simulink model "Template_v4_1_0_2024b_Jetson"  (R2024b)
settings: Solver=ode4  StartTime=0.0  StopTime=tsim  FixedStep=baseRate  RelTol=1e-6  AbsTol=1e-6
undefined symbols (not defined in the file): a1, a2, a3, b0, b1, b2, b3, baseRate, dataRate, DiscIntNeverNeededParam, drop_states_ARM, drop_states_BLACK, drop_states_BLUE, drop_states_RED, F_black_X_nominal, F_black_Y_nominal, F_blue_X_nominal, F_blue_Y_nominal, F_red_X_nominal, F_red_Y_nominal, F_thrusters_BLACK, F_thrusters_BLUE, F_thrusters_RED, Gamma1_el, Gamma1_sh, Gamma1_wr, Gamma2_el, Gamma2_sh, Gamma2_wr, Gamma3_el, Gamma3_sh, Gamma3_wr, Gamma4_el, Gamma4_sh, Gamma4_wr, Gamma5_el, Gamma5_sh, Gamma5_wr, Gamma6_el, Gamma6_sh, Gamma6_wr, home_states_BLACK, home_states_BLUE, home_states_RED, IBLACK, IBLUE, IDIST, IEE, init_states_BLACK, init_states_BLUE, init_states_RED, IPROX, IRED, K_BLACK, K_BLUE, K_RED, Kd_elarm, Kd_sharm, Kd_tb, Kd_tblue ... (+49)
libraries: simulink x30, dspsigops x12, nvidiaSharedBlocks x12, MainLibrary x5, dspinverses x3, nvidiaIMUSensorslib x1
(part 2 of 7)

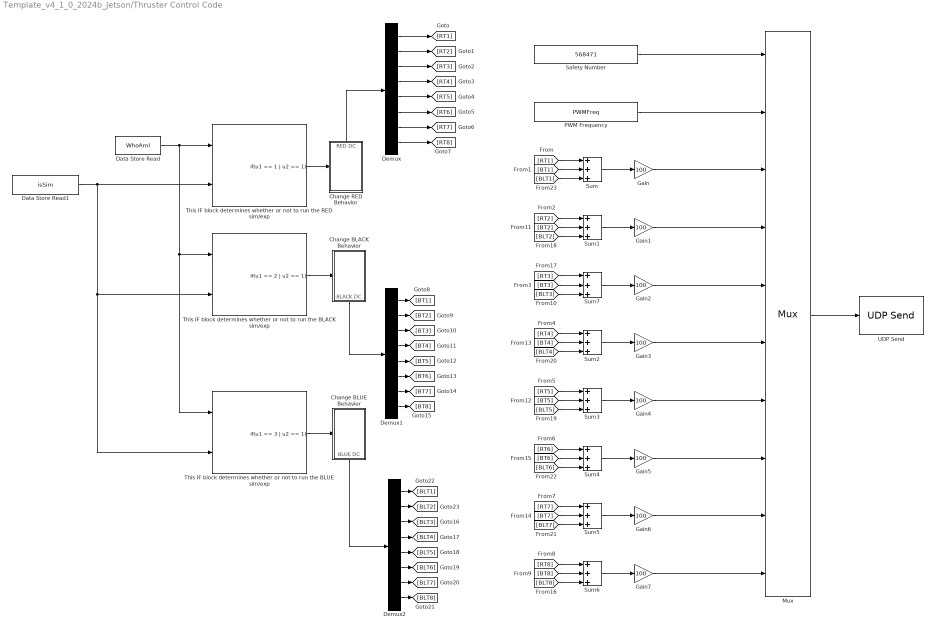
== system Template_v4_1_0_2024b_Jetson/Thruster Control Code ==
  Change BLACK Behavior : Subsystem  TreatAsAtomicUnit=on
  Change BLUE Behavior : Subsystem  TreatAsAtomicUnit=on
  Change RED Behavior : Subsystem  TreatAsAtomicUnit=on
  Data Store Read : DataStoreRead  DataStoreName=WhoAmI  IndexOptions=Index vector (dialog)  Indices=1  OutputSizes=1
  Data Store Read1 : DataStoreRead  DataStoreName=isSim  IndexOptions=Index vector (dialog)  Indices=1  OutputSizes=1
  Demux : Demux  Outputs=8
  Demux1 : Demux  Outputs=8
  Demux2 : Demux  Outputs=8
  Gain{,1..7} (8 alike) : Gain  Gain=100
  Mux : Mux  Inputs=10
  PWM Frequency : Constant  Value=PWMFreq
  Safety Number : Constant  Value=568471
  Sum{,1..7} (8 alike) : Sum  Inputs=+++
  This IF block determines whether or not to run the BLACK sim/exp : If  NumInputs=2  IfExpression=u1 == 2 | u2 == 1  ShowElse=off
  This IF block determines whether or not to run the BLUE sim/exp : If  NumInputs=2  IfExpression=u1 == 3 | u2 == 1  ShowElse=off
  "This IF block determines whether or not to run the RED sim/exp " : If  NumInputs=2  IfExpression=u1 == 1 | u2 == 1  ShowElse=off
  UDP Send : nvidiaSharedBlocks/UDP Send  remoteURL='127.0.0.1'  remotePort=48291  localURL='0.0.0.0'  localPortSource=Automatically determine  localPort=-1  sampletime=-1  blockPlatform=NVIDIA  separateLengthPort=0
      settings: LibrarySourceBlock=nvidiaNetworklib/UDP Send
  wires:
  Data Store Read1/1 -> This IF block determines whether or not to run the BLACK sim/exp/2, This IF block determines whether or not to run the BLUE sim/exp/2, "This IF block determines whether or not to run the RED sim/exp "/2
  "This IF block determines whether or not to run the RED sim/exp "/1 -> Change RED Behavior/Action
  This IF block determines whether or not to run the BLACK sim/exp/1 -> Change BLACK Behavior/Action
  Change RED Behavior/1(RED DC) -> Demux/1
  Demux/1 -> [RT1]
  Demux/2 -> [RT2]
  Demux/3 -> [RT3]
  Demux/4 -> [RT4]
  Demux/5 -> [RT5]
  Demux/6 -> [RT6]
  Demux/7 -> [RT7]
  Demux/8 -> [RT8]
  Demux1/5 -> [BT5]
  Demux1/4 -> [BT4]
  Demux1/1 -> [BT1]
  Demux1/8 -> [BT8]
  Demux1/2 -> [BT2]
  Demux1/7 -> [BT7]
  Demux1/6 -> [BT6]
  Demux1/3 -> [BT3]
  Change BLACK Behavior/1(BLACK DC) -> Demux1/1
  Data Store Read/1 -> This IF block determines whether or not to run the BLUE sim/exp/1, This IF block determines whether or not to run the BLACK sim/exp/1, "This IF block determines whether or not to run the RED sim/exp "/1
  This IF block determines whether or not to run the BLUE sim/exp/1 -> Change BLUE Behavior/Action
  Demux2/5 -> [BLT5]
  Demux2/8 -> [BLT8]
  Demux2/7 -> [BLT7]
  Demux2/2 -> [BLT2]
  Change BLUE Behavior/1(BLUE DC) -> Demux2/1
  Demux2/1 -> [BLT1]
  Demux2/4 -> [BLT4]
  Demux2/3 -> [BLT3]
  Demux2/6 -> [BLT6]
  [BT5] -> Sum3/2
  [RT4] -> Sum2/1
  Sum3/1 -> Gain4/1
  [RT2] -> Sum1/1
  [BLT4] -> Sum2/3
  [BT3] -> Sum7/2
  [RT5] -> Sum3/1
  PWM Frequency/1 -> Mux/2
  Gain3/1 -> Mux/6
  [BT8] -> Sum6/2
  Gain7/1 -> Mux/10
  Sum6/1 -> Gain7/1
  Sum7/1 -> Gain2/1
  [BT4] -> Sum2/2
  [RT7] -> Sum5/1
  [BLT3] -> Sum7/3
  Gain1/1 -> Mux/4
  Gain/1 -> Mux/3
  [BLT5] -> Sum3/3
  Sum1/1 -> Gain1/1
  Sum2/1 -> Gain3/1
  Gain4/1 -> Mux/7
  [BLT6] -> Sum4/3
  [BT6] -> Sum4/2
  [BT2] -> Sum1/2
  [BLT2] -> Sum1/3
  [RT1] -> Sum/1
  Sum/1 -> Gain/1
  [BT7] -> Sum5/2
  Gain6/1 -> Mux/9
  [BLT7] -> Sum5/3
  [RT8] -> Sum6/1
  [RT6] -> Sum4/1
  Mux/1 -> UDP Send/1
  [BLT8] -> Sum6/3
  [BT1] -> Sum/2
  Sum5/1 -> Gain6/1
  Gain5/1 -> Mux/8
  Sum4/1 -> Gain5/1
  [BLT1] -> Sum/3
  Safety Number/1 -> Mux/1
  [RT3] -> Sum7/1
  Gain2/1 -> Mux/5

== system Template_v4_1_0_2024b_Jetson/1 - Experiment Logic/Phase #0: Synchronization ==
  note: Setting the RED thrusters to OFF.
  note: Setting the PUCKS for ALL to OFF.
  note: DISABLE ARM Path Planning.
  note: Setting the BLACK thrusters to OFF.
  note: Setting the BLUE thrusters to OFF.
  note: DISABLE RED Path Planning.
  note: DISABLE BLACK Path Planning.
  note: DISABLE BLUE Path Planning.
  note: DISABLE ARM Control.
  Action Port : ActionPort  ActionPortLabel=if(u1 < u2)
  Constant{1..8} (8 alike) : Constant  Value=0
  Data Store Write : DataStoreWrite  DataStoreName=RED_Control_Law_Enabler  IndexOptions=Index vector (dialog)  Indices=1  OutputSizes=1
  Data Store Write1 : DataStoreWrite  DataStoreName=RED_Logger  IndexOptions=Index vector (dialog)  Indices=1  OutputSizes=1
  Data Store Write2 : DataStoreWrite  DataStoreName=BLACK_Control_Law_Enabler  IndexOptions=Index vector (dialog)  Indices=1  OutputSizes=1
  Data Store Write3 : DataStoreWrite  DataStoreName=BLUE_Control_Law_Enabler  IndexOptions=Index vector (dialog)  Indices=1  OutputSizes=1
  Data Store Write4 : DataStoreWrite  DataStoreName=Float_State  IndexOptions=Index vector (dialog)  Indices=1  OutputSizes=1
  Data Store Write5 : DataStoreWrite  DataStoreName=BLUE_Path_Planner_Selection  IndexOptions=Index vector (dialog)  Indices=1  OutputSizes=1
  Data Store Write6 : DataStoreWrite  DataStoreName=BLACK_Path_Planner_Selection  IndexOptions=Index vector (dialog)  Indices=1  OutputSizes=1
  Data Store Write7 : DataStoreWrite  DataStoreName=RED_Path_Planner_Selection  IndexOptions=Index vector (dialog)  Indices=1  OutputSizes=1
  Data Store Write8 : DataStoreWrite  DataStoreName=ARM_Path_Planner_Selection  IndexOptions=Index vector (dialog)  Indices=1  OutputSizes=1
  Data Store Write9 : DataStoreWrite  DataStoreName=ARM_Control_Law_Enabler  IndexOptions=Index vector (dialog)  Indices=1  OutputSizes=1
  Puck State : Constant  Value=0
  String Constant : StringConstant  String="\"Chaser: Running Phase 0\""
  wires:
  Constant4/1 -> Data Store Write8/1
  Puck State/1 -> Data Store Write4/1
  Constant5/1 -> Data Store Write/1
  Constant1/1 -> Data Store Write2/1
  Constant2/1 -> Data Store Write3/1
  Constant3/1 -> Data Store Write7/1
  Constant6/1 -> Data Store Write6/1
  Constant7/1 -> Data Store Write5/1
  Constant8/1 -> Data Store Write9/1
  String Constant/1 -> Data Store Write1/1

== system Template_v4_1_0_2024b_Jetson/1 - Experiment Logic/Phase #1: Start Floating  ==
  note: DISABLE ARM Control.
  note: Setting the BLACK thrusters to OFF.
  note: Setting the PUCKS for ALL to OFF.
  note: DISABLE RED Path Planning.
  note: Setting the RED thrusters to OFF.
  note: Setting the BLUE thrusters to OFF.
  note: DISABLE ARM Path Planning.
  note: DISABLE BLACK Path Planning.
  note: DISABLE BLUE Path Planning.
  Action Port : ActionPort  ActionPortLabel=elseif((u1 < u3 & u1 >= u2))
  Constant{1..8} (8 alike) : Constant  Value=0
  Data Store Write : DataStoreWrite  DataStoreName=RED_Control_Law_Enabler  IndexOptions=Index vector (dialog)  Indices=1  OutputSizes=1
  Data Store Write1 : DataStoreWrite  DataStoreName=RED_Logger  IndexOptions=Index vector (dialog)  Indices=1  OutputSizes=1
  Data Store Write2 : DataStoreWrite  DataStoreName=BLACK_Control_Law_Enabler  IndexOptions=Index vector (dialog)  Indices=1  OutputSizes=1
  Data Store Write3 : DataStoreWrite  DataStoreName=BLUE_Control_Law_Enabler  IndexOptions=Index vector (dialog)  Indices=1  OutputSizes=1
  Data Store Write4 : DataStoreWrite  DataStoreName=Float_State  IndexOptions=Index vector (dialog)  Indices=1  OutputSizes=1
  Data Store Write5 : DataStoreWrite  DataStoreName=BLUE_Path_Planner_Selection  IndexOptions=Index vector (dialog)  Indices=1  OutputSizes=1
  Data Store Write6 : DataStoreWrite  DataStoreName=BLACK_Path_Planner_Selection  IndexOptions=Index vector (dialog)  Indices=1  OutputSizes=1
  Data Store Write7 : DataStoreWrite  DataStoreName=RED_Path_Planner_Selection  IndexOptions=Index vector (dialog)  Indices=1  OutputSizes=1
  Data Store Write8 : DataStoreWrite  DataStoreName=ARM_Path_Planner_Selection  IndexOptions=Index vector (dialog)  Indices=1  OutputSizes=1
  Data Store Write9 : DataStoreWrite  DataStoreName=ARM_Control_Law_Enabler  IndexOptions=Index vector (dialog)  Indices=1  OutputSizes=1
  Puck State : Constant
  String Constant : StringConstant  String="\"Chaser: Running Phase 1\""
  wires:
  Constant7/1 -> Data Store Write5/1
  Constant2/1 -> Data Store Write3/1
  Constant6/1 -> Data Store Write6/1
  Puck State/1 -> Data Store Write4/1
  Constant1/1 -> Data Store Write2/1
  Constant5/1 -> Data Store Write/1
  Constant3/1 -> Data Store Write7/1
  Constant8/1 -> Data Store Write9/1
  Constant4/1 -> Data Store Write8/1
  String Constant/1 -> Data Store Write1/1

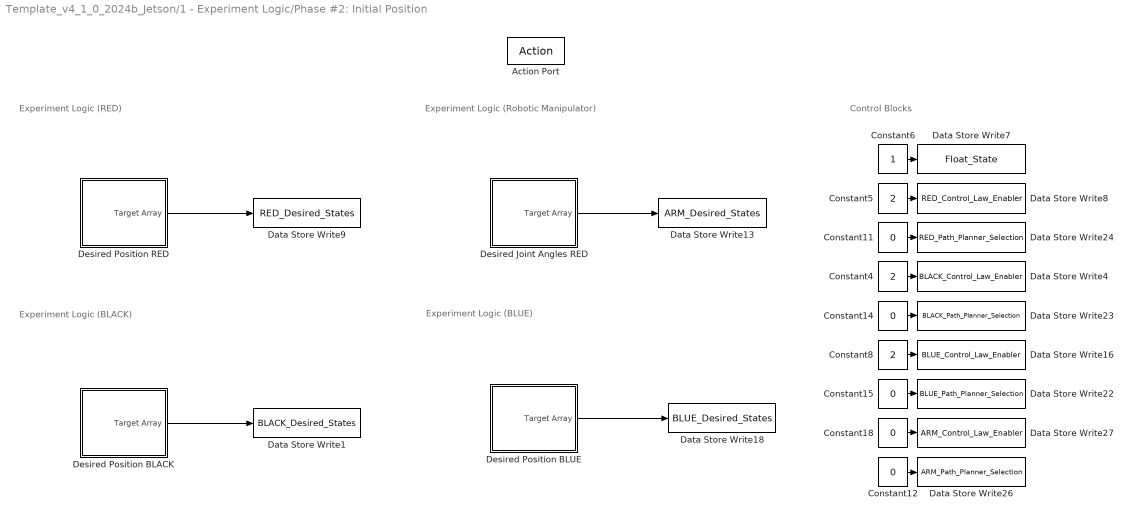
== system Template_v4_1_0_2024b_Jetson/1 - Experiment Logic/Phase #2: Initial Position ==
  note: Experiment Logic (BLACK)
  note: Control Blocks
  note: Experiment Logic (RED)
  note: Experiment Logic (Robotic Manipulator)
  note: Experiment Logic (BLUE)
  Action Port : ActionPort  ActionPortLabel=elseif((u1 < u4 & u1 >= u3))
  Constant{11..12,14..15,18} (5 alike) : Constant  Value=0
  Constant4 : Constant  Value=2
  Constant5 : Constant  Value=2
  Constant6 : Constant
  Constant8 : Constant  Value=2
  Data Store Write1 : DataStoreWrite  DataStoreName=BLACK_Desired_States  IndexOptions=Index vector (dialog)  Indices=1  OutputSizes=1
  Data Store Write13 : DataStoreWrite  DataStoreName=ARM_Desired_States  IndexOptions=Index vector (dialog)  Indices=1  OutputSizes=1
  Data Store Write16 : DataStoreWrite  DataStoreName=BLUE_Control_Law_Enabler  IndexOptions=Index vector (dialog)  Indices=1  OutputSizes=1
  Data Store Write18 : DataStoreWrite  DataStoreName=BLUE_Desired_States  IndexOptions=Index vector (dialog)  Indices=1  OutputSizes=1
  Data Store Write22 : DataStoreWrite  DataStoreName=BLUE_Path_Planner_Selection  IndexOptions=Index vector (dialog)  Indices=1  OutputSizes=1
  Data Store Write23 : DataStoreWrite  DataStoreName=BLACK_Path_Planner_Selection  IndexOptions=Index vector (dialog)  Indices=1  OutputSizes=1
  Data Store Write24 : DataStoreWrite  DataStoreName=RED_Path_Planner_Selection  IndexOptions=Index vector (dialog)  Indices=1  OutputSizes=1
  Data Store Write26 : DataStoreWrite  DataStoreName=ARM_Path_Planner_Selection  IndexOptions=Index vector (dialog)  Indices=1  OutputSizes=1
  Data Store Write27 : DataStoreWrite  DataStoreName=ARM_Control_Law_Enabler  IndexOptions=Index vector (dialog)  Indices=1  OutputSizes=1
  Data Store Write4 : DataStoreWrite  DataStoreName=BLACK_Control_Law_Enabler  IndexOptions=Index vector (dialog)  Indices=1  OutputSizes=1
  Data Store Write7 : DataStoreWrite  DataStoreName=Float_State  IndexOptions=Index vector (dialog)  Indices=1  OutputSizes=1
  Data Store Write8 : DataStoreWrite  DataStoreName=RED_Control_Law_Enabler  IndexOptions=Index vector (dialog)  Indices=1  OutputSizes=1
  Data Store Write9 : DataStoreWrite  DataStoreName=RED_Desired_States  IndexOptions=Index vector (dialog)  Indices=1  OutputSizes=1
  Desired Joint Angles RED : Subsystem
  Desired Position BLACK : Subsystem
  Desired Position BLUE : Subsystem
  Desired Position RED : Subsystem
  wires:
  Constant4/1 -> Data Store Write4/1
  Constant8/1 -> Data Store Write16/1
  Desired Position BLACK/1(Target Array) -> Data Store Write1/1
  Constant5/1 -> Data Store Write8/1
  Desired Position RED/1(Target Array) -> Data Store Write9/1
  Constant6/1 -> Data Store Write7/1
  Desired Position BLUE/1(Target Array) -> Data Store Write18/1
  Constant11/1 -> Data Store Write24/1
  Constant14/1 -> Data Store Write23/1
  Constant15/1 -> Data Store Write22/1
  Desired Joint Angles RED/1(Target Array) -> Data Store Write13/1
  Constant18/1 -> Data Store Write27/1
  Constant12/1 -> Data Store Write26/1

== system Template_v4_1_0_2024b_Jetson/1 - Experiment Logic/Phase #3: Experiment ==
  Action Port : ActionPort  ActionPortLabel=elseif( (u1 < u5 & u1 >= u4))
  Constant1 : Constant  Value=Phase3_SubPhase2_End  SampleTime=-1
  Constant2 : Constant  Value=Phase3_SubPhase3_End  SampleTime=-1
  Constant3 : Constant  Value=Phase3_SubPhase4_End  SampleTime=-1
  Constant4 : Constant  Value=Phase3_SubPhase1_End  SampleTime=-1
  Experiment Sub-Phases : If  NumInputs=5  IfExpression=u1 < u2  ElseIfExpressions=(u1 < u3 & u1 >= u2),(u1 < u4 & u1 >= u3), (u1 < u5 & u1 >= u4)  ShowElse=off
  Sub-Phase #1 : Subsystem  TreatAsAtomicUnit=on
  "Sub-Phase #2 " : Subsystem  TreatAsAtomicUnit=on
  "Sub-Phase #3 " : Subsystem  TreatAsAtomicUnit=on
  Sub-Phase #4 : Subsystem  TreatAsAtomicUnit=on
  Universal_Time : DataStoreRead  DataStoreName=Univ_Time  IndexOptions=Index vector (dialog)  Indices=1  OutputSizes=1
  wires:
  Experiment Sub-Phases/3 -> "Sub-Phase #3 "/Action
  Experiment Sub-Phases/4 -> Sub-Phase #4/Action
  Constant3/1 -> Experiment Sub-Phases/5
  Constant2/1 -> Experiment Sub-Phases/4
  Experiment Sub-Phases/1 -> Sub-Phase #1/Action
  Experiment Sub-Phases/2 -> "Sub-Phase #2 "/Action
  Constant1/1 -> Experiment Sub-Phases/3
  Constant4/1 -> Experiment Sub-Phases/2
  Universal_Time/1 -> Experiment Sub-Phases/1

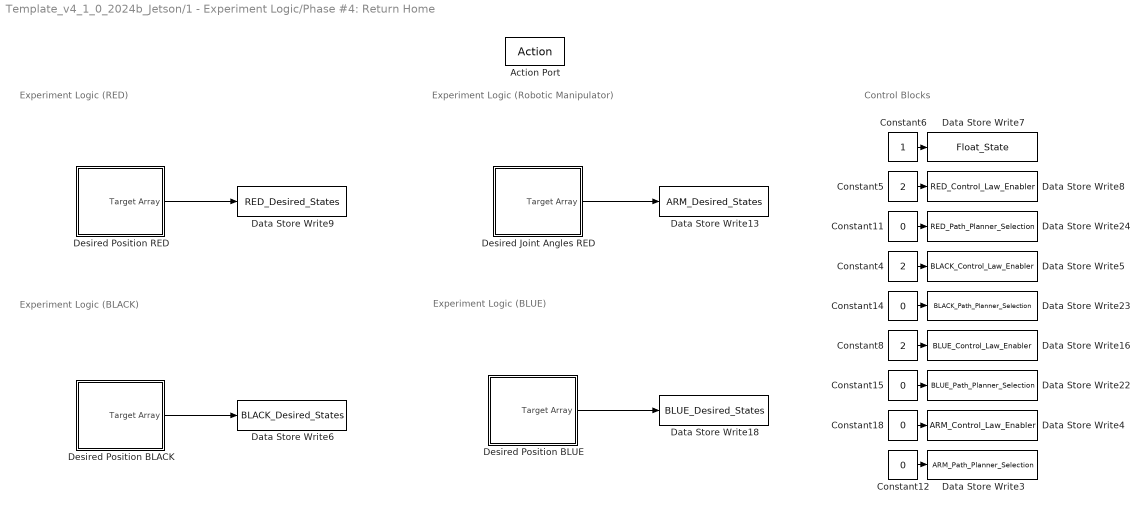
== system Template_v4_1_0_2024b_Jetson/1 - Experiment Logic/Phase #4: Return Home ==
  note: Experiment Logic (BLACK)
  note: Experiment Logic (Robotic Manipulator)
  note: Experiment Logic (BLUE)
  note: Experiment Logic (RED)
  note: Control Blocks
  Action Port : ActionPort  ActionPortLabel=elseif((u1 < u6 & u1 >= u5))
  Constant{11..12,14..15,18} (5 alike) : Constant  Value=0
  Constant4 : Constant  Value=2
  Constant5 : Constant  Value=2
  Constant6 : Constant
  Constant8 : Constant  Value=2
  Data Store Write13 : DataStoreWrite  DataStoreName=ARM_Desired_States  IndexOptions=Index vector (dialog)  Indices=1  OutputSizes=1
  Data Store Write16 : DataStoreWrite  DataStoreName=BLUE_Control_Law_Enabler  IndexOptions=Index vector (dialog)  Indices=1  OutputSizes=1
  Data Store Write18 : DataStoreWrite  DataStoreName=BLUE_Desired_States  IndexOptions=Index vector (dialog)  Indices=1  OutputSizes=1
  Data Store Write22 : DataStoreWrite  DataStoreName=BLUE_Path_Planner_Selection  IndexOptions=Index vector (dialog)  Indices=1  OutputSizes=1
  Data Store Write23 : DataStoreWrite  DataStoreName=BLACK_Path_Planner_Selection  IndexOptions=Index vector (dialog)  Indices=1  OutputSizes=1
  Data Store Write24 : DataStoreWrite  DataStoreName=RED_Path_Planner_Selection  IndexOptions=Index vector (dialog)  Indices=1  OutputSizes=1
  Data Store Write3 : DataStoreWrite  DataStoreName=ARM_Path_Planner_Selection  IndexOptions=Index vector (dialog)  Indices=1  OutputSizes=1
  Data Store Write4 : DataStoreWrite  DataStoreName=ARM_Control_Law_Enabler  IndexOptions=Index vector (dialog)  Indices=1  OutputSizes=1
  Data Store Write5 : DataStoreWrite  DataStoreName=BLACK_Control_Law_Enabler  IndexOptions=Index vector (dialog)  Indices=1  OutputSizes=1
  Data Store Write6 : DataStoreWrite  DataStoreName=BLACK_Desired_States  IndexOptions=Index vector (dialog)  Indices=1  OutputSizes=1
  Data Store Write7 : DataStoreWrite  DataStoreName=Float_State  IndexOptions=Index vector (dialog)  Indices=1  OutputSizes=1
  Data Store Write8 : DataStoreWrite  DataStoreName=RED_Control_Law_Enabler  IndexOptions=Index vector (dialog)  Indices=1  OutputSizes=1
  Data Store Write9 : DataStoreWrite  DataStoreName=RED_Desired_States  IndexOptions=Index vector (dialog)  Indices=1  OutputSizes=1
  Desired Joint Angles RED : Subsystem
  Desired Position BLACK : Subsystem
  Desired Position BLUE : Subsystem
  Desired Position RED : Subsystem
  wires:
  Desired Position RED/1(Target Array) -> Data Store Write9/1
  Desired Position BLACK/1(Target Array) -> Data Store Write6/1
  Desired Position BLUE/1(Target Array) -> Data Store Write18/1
  Constant12/1 -> Data Store Write3/1
  Constant18/1 -> Data Store Write4/1
  Constant6/1 -> Data Store Write7/1
  Constant15/1 -> Data Store Write22/1
  Constant14/1 -> Data Store Write23/1
  Constant5/1 -> Data Store Write8/1
  Constant11/1 -> Data Store Write24/1
  Constant8/1 -> Data Store Write16/1
  Constant4/1 -> Data Store Write5/1
  Desired Joint Angles RED/1(Target Array) -> Data Store Write13/1

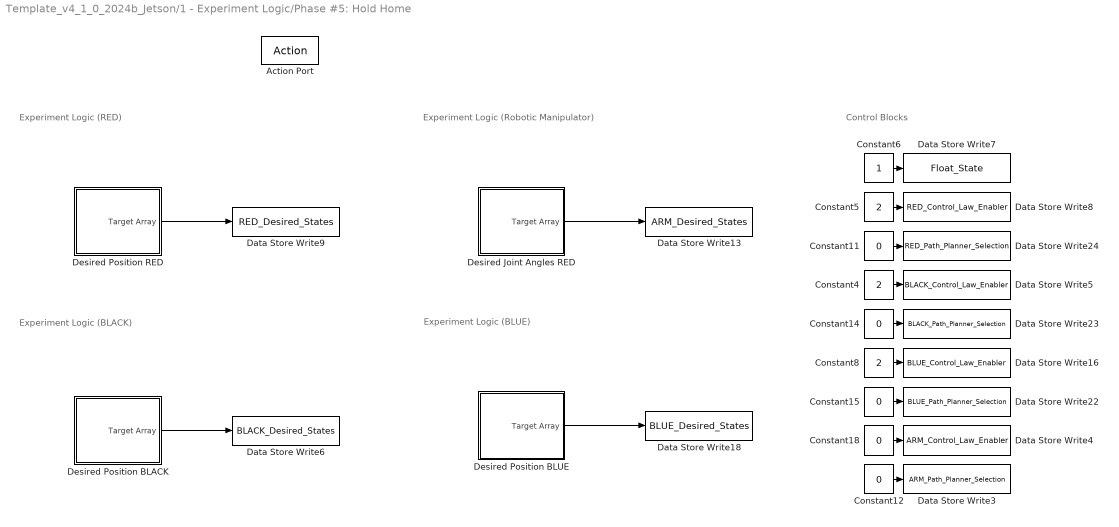
== system Template_v4_1_0_2024b_Jetson/1 - Experiment Logic/Phase #5: Hold Home ==
  note: Experiment Logic (BLUE)
  note: Experiment Logic (BLACK)
  note: Control Blocks
  note: Experiment Logic (RED)
  note: Experiment Logic (Robotic Manipulator)
  Action Port : ActionPort  ActionPortLabel=elseif( (u1 < u7 & u1 >= u6) )
  Constant{11..12,14..15,18} (5 alike) : Constant  Value=0
  Constant4 : Constant  Value=2
  Constant5 : Constant  Value=2
  Constant6 : Constant
  Constant8 : Constant  Value=2
  Data Store Write13 : DataStoreWrite  DataStoreName=ARM_Desired_States  IndexOptions=Index vector (dialog)  Indices=1  OutputSizes=1
  Data Store Write16 : DataStoreWrite  DataStoreName=BLUE_Control_Law_Enabler  IndexOptions=Index vector (dialog)  Indices=1  OutputSizes=1
  Data Store Write18 : DataStoreWrite  DataStoreName=BLUE_Desired_States  IndexOptions=Index vector (dialog)  Indices=1  OutputSizes=1
  Data Store Write22 : DataStoreWrite  DataStoreName=BLUE_Path_Planner_Selection  IndexOptions=Index vector (dialog)  Indices=1  OutputSizes=1
  Data Store Write23 : DataStoreWrite  DataStoreName=BLACK_Path_Planner_Selection  IndexOptions=Index vector (dialog)  Indices=1  OutputSizes=1
  Data Store Write24 : DataStoreWrite  DataStoreName=RED_Path_Planner_Selection  IndexOptions=Index vector (dialog)  Indices=1  OutputSizes=1
  Data Store Write3 : DataStoreWrite  DataStoreName=ARM_Path_Planner_Selection  IndexOptions=Index vector (dialog)  Indices=1  OutputSizes=1
  Data Store Write4 : DataStoreWrite  DataStoreName=ARM_Control_Law_Enabler  IndexOptions=Index vector (dialog)  Indices=1  OutputSizes=1
  Data Store Write5 : DataStoreWrite  DataStoreName=BLACK_Control_Law_Enabler  IndexOptions=Index vector (dialog)  Indices=1  OutputSizes=1
  Data Store Write6 : DataStoreWrite  DataStoreName=BLACK_Desired_States  IndexOptions=Index vector (dialog)  Indices=1  OutputSizes=1
  Data Store Write7 : DataStoreWrite  DataStoreName=Float_State  IndexOptions=Index vector (dialog)  Indices=1  OutputSizes=1
  Data Store Write8 : DataStoreWrite  DataStoreName=RED_Control_Law_Enabler  IndexOptions=Index vector (dialog)  Indices=1  OutputSizes=1
  Data Store Write9 : DataStoreWrite  DataStoreName=RED_Desired_States  IndexOptions=Index vector (dialog)  Indices=1  OutputSizes=1
  Desired Joint Angles RED : Subsystem
  Desired Position BLACK : Subsystem
  Desired Position BLUE : Subsystem
  Desired Position RED : Subsystem
  wires:
  Desired Position RED/1(Target Array) -> Data Store Write9/1
  Desired Position BLACK/1(Target Array) -> Data Store Write6/1
  Desired Position BLUE/1(Target Array) -> Data Store Write18/1
  Constant12/1 -> Data Store Write3/1
  Constant18/1 -> Data Store Write4/1
  Constant6/1 -> Data Store Write7/1
  Constant15/1 -> Data Store Write22/1
  Constant14/1 -> Data Store Write23/1
  Constant5/1 -> Data Store Write8/1
  Constant11/1 -> Data Store Write24/1
  Constant8/1 -> Data Store Write16/1
  Constant4/1 -> Data Store Write5/1
  Desired Joint Angles RED/1(Target Array) -> Data Store Write13/1

== system Template_v4_1_0_2024b_Jetson/1 - Experiment Logic/Phase #6: Clean Shutdown ==
  note: DISABLE ARM Control.
  note: Setting the BLACK thrusters to OFF.
  note: Setting the PUCKS for ALL to OFF.
  note: DISABLE RED Path Planning.
  note: Setting the RED thrusters to OFF.
  note: Setting the BLUE thrusters to OFF.
  note: DISABLE ARM Path Planning.
  note: DISABLE BLACK Path Planning.
  note: DISABLE BLUE Path Planning.
  Action Port : ActionPort  ActionPortLabel=elseif((u1 >= u7))
  Constant{1..8} (8 alike) : Constant  Value=0
  Data Store Write : DataStoreWrite  DataStoreName=RED_Control_Law_Enabler  IndexOptions=Index vector (dialog)  Indices=1  OutputSizes=1
  Data Store Write2 : DataStoreWrite  DataStoreName=BLACK_Control_Law_Enabler  IndexOptions=Index vector (dialog)  Indices=1  OutputSizes=1
  Data Store Write3 : DataStoreWrite  DataStoreName=BLUE_Control_Law_Enabler  IndexOptions=Index vector (dialog)  Indices=1  OutputSizes=1
  Data Store Write4 : DataStoreWrite  DataStoreName=Float_State  IndexOptions=Index vector (dialog)  Indices=1  OutputSizes=1
  Data Store Write5 : DataStoreWrite  DataStoreName=BLUE_Path_Planner_Selection  IndexOptions=Index vector (dialog)  Indices=1  OutputSizes=1
  Data Store Write6 : DataStoreWrite  DataStoreName=BLACK_Path_Planner_Selection  IndexOptions=Index vector (dialog)  Indices=1  OutputSizes=1
  Data Store Write7 : DataStoreWrite  DataStoreName=RED_Path_Planner_Selection  IndexOptions=Index vector (dialog)  Indices=1  OutputSizes=1
  Data Store Write8 : DataStoreWrite  DataStoreName=ARM_Path_Planner_Selection  IndexOptions=Index vector (dialog)  Indices=1  OutputSizes=1
  Data Store Write9 : DataStoreWrite  DataStoreName=ARM_Control_Law_Enabler  IndexOptions=Index vector (dialog)  Indices=1  OutputSizes=1
  Puck State : Constant  Value=0
  wires:
  Constant7/1 -> Data Store Write5/1
  Constant2/1 -> Data Store Write3/1
  Constant6/1 -> Data Store Write6/1
  Puck State/1 -> Data Store Write4/1
  Constant1/1 -> Data Store Write2/1
  Constant5/1 -> Data Store Write/1
  Constant3/1 -> Data Store Write7/1
  Constant8/1 -> Data Store Write9/1
  Constant4/1 -> Data Store Write8/1

== system Template_v4_1_0_2024b_Jetson/2 - Guidance/Custom PPL (ARM) ==
  Action Port : ActionPort  ActionPortLabel=if(u1 == 2)
  Desired Position : Subsystem
  Path : Outport
  wires:
  Desired Position/1(Position Array) -> Path/1

== system Template_v4_1_0_2024b_Jetson/2 - Guidance/Custom PPL (BLACK) ==
  Action Port : ActionPort  ActionPortLabel=elseif(u1 == 2)
  Desired Position : Subsystem
  Path : Outport
  wires:
  Desired Position/1(Position Array) -> Path/1

== system Template_v4_1_0_2024b_Jetson/2 - Guidance/Custom PPL (BLUE) ==
  Action Port : ActionPort  ActionPortLabel=if(u1 == 2)
  Desired Position : Subsystem
  Path : Outport
  wires:
  Desired Position/1(Position Array) -> Path/1

== system Template_v4_1_0_2024b_Jetson/2 - Guidance/Custom PPL (RED) ==
  Action Port : ActionPort  ActionPortLabel=elseif(u1 == 2)
  Desired Position : Subsystem
  Path : Outport
  wires:
  Desired Position/1(Position Array) -> Path/1

== system Template_v4_1_0_2024b_Jetson/2 - Guidance/Default APF PPL (BLACK) ==
  Action Port : ActionPort  ActionPortLabel=if(u1 == 1 )
  Angular Gain : Constant  Value=200
  Attractive Gain : Constant  Value=200
  Current Position RED : Subsystem
  Influence Range : Constant
  MATLAB Function : MATLAB Function  TreatAsAtomicUnit=on
  Obstacles : Subsystem
  RED_Px : DataStoreRead  DataStoreName=BLACK_Desired_States  IndexOptions=Index vector (dialog)  Indices=1  OutputSizes=1
  Repulsive Gain : Constant  Value=5
  Reshape : Reshape  OutputDimensionality=Row vector (2-D)
  Reshape1 : Reshape  OutputDimensionality=Row vector (2-D)
  Path : Outport
  wires:
  Obstacles/1(Obstacle Positions) -> MATLAB Function/3(obstacles)
  MATLAB Function/1(currentPosition) -> Path/1
  Reshape/1 -> MATLAB Function/1(desiredPosition)
  Angular Gain/1 -> MATLAB Function/7(angularGain)
  RED_Px/1 -> Reshape/1
  Attractive Gain/1 -> MATLAB Function/4(attractiveGain)
  Repulsive Gain/1 -> MATLAB Function/5(repulsiveGain)
  Reshape1/1 -> MATLAB Function/2("currentPosition ")
  Influence Range/1 -> MATLAB Function/6(influenceRange)
  Current Position RED/1(Position Array) -> Reshape1/1

== system Template_v4_1_0_2024b_Jetson/2 - Guidance/Default APF PPL (RED) ==
  Action Port : ActionPort  ActionPortLabel=if(u1 == 1 )
  Angular Gain : Constant  Value=200
  Attractive Gain : Constant  Value=200
  Current Position RED : Subsystem
  Influence Range : Constant
  MATLAB Function : MATLAB Function  TreatAsAtomicUnit=on
  Obstacles : Subsystem
  RED_Px : DataStoreRead  DataStoreName=RED_Desired_States  IndexOptions=Index vector (dialog)  Indices=1  OutputSizes=1
  Repulsive Gain : Constant  Value=5
  Reshape : Reshape  OutputDimensionality=Row vector (2-D)
  Reshape1 : Reshape  OutputDimensionality=Row vector (2-D)
  Path : Outport
  wires:
  MATLAB Function/1(currentPosition) -> Path/1
  Reshape/1 -> MATLAB Function/1(desiredPosition)
  Reshape1/1 -> MATLAB Function/2("currentPosition ")
  Current Position RED/1(Position Array) -> Reshape1/1
  Obstacles/1(Obstacle Positions) -> MATLAB Function/3(obstacles)
  RED_Px/1 -> Reshape/1
  Attractive Gain/1 -> MATLAB Function/4(attractiveGain)
  Angular Gain/1 -> MATLAB Function/7(angularGain)
  Influence Range/1 -> MATLAB Function/6(influenceRange)
  Repulsive Gain/1 -> MATLAB Function/5(repulsiveGain)

== system Template_v4_1_0_2024b_Jetson/2 - Guidance/Disable PPL (ARM) ==
  Action Port : ActionPort  ActionPortLabel=else
  Desired Position : Subsystem
  Path : Outport
  wires:
  Desired Position/1(Position Array) -> Path/1

== system Template_v4_1_0_2024b_Jetson/2 - Guidance/Disable PPL (BLACK) ==
  Action Port : ActionPort  ActionPortLabel=else
  Desired Position : Subsystem
  Path : Outport
  wires:
  Desired Position/1(Position Array) -> Path/1

== system Template_v4_1_0_2024b_Jetson/2 - Guidance/Disable PPL (BLUE) ==
  Action Port : ActionPort  ActionPortLabel=else
  Desired Position : Subsystem
  Path : Outport
  wires:
  Desired Position/1(Position Array) -> Path/1

== system Template_v4_1_0_2024b_Jetson/2 - Guidance/Disable PPL (RED) ==
  Action Port : ActionPort  ActionPortLabel=else
  Desired Position : Subsystem
  Path : Outport
  wires:
  Desired Position/1(Position Array) -> Path/1

== system Template_v4_1_0_2024b_Jetson/3 - Control/Custom Control (ARM) ==
  Action Port : ActionPort  ActionPortLabel=elseif(u1 == 2)
  Mux : Mux  Inputs=3
  Zero : Constant  Value=0  OutDataTypeStr=Inherit: Inherit via back propagation
  u : Outport
  wires:
  Mux/1 -> u/1
  Zero/1 -> Mux/3, Mux/1, Mux/2

== system Template_v4_1_0_2024b_Jetson/3 - Control/Custom Control (RED) ==
  Action Port : ActionPort  ActionPortLabel=elseif( u1 == 3)
  Mux : Mux  Inputs=3
  Zero : Constant  Value=0  OutDataTypeStr=Inherit: Inherit via back propagation
  u : Outport
  wires:
  Zero/1 -> Mux/3, Mux/1, Mux/2
  Mux/1 -> u/1

== system Template_v4_1_0_2024b_Jetson/3 - Control/Default LQR Control (BLACK) ==
  Action Port : ActionPort  ActionPortLabel=elseif(u1 == 2)
  Calculate Error : Subsystem
  Constant2 : Constant  Value=-K_BLACK
  Data Store Read1 : DataStoreRead  DataStoreName=BLACK_Path  IndexOptions=Index vector (dialog)  Indices=1  OutputSizes=1
  Data Store Read13 : DataStoreRead  DataStoreName=BLACK_Measured_States  IndexOptions=Index vector (dialog)  Indices=1  OutputSizes=1
  Demux : Demux  Outputs=[1,1,1,1,1,1,3]
  Demux1 : Demux  Outputs=3
  Discrete Derivative : simulink/Discrete/Discrete Derivative  gainval=1.0  ICPrevScaledInput=0.0  OutMin=[]  OutMax=[]  OutDataType=fixdt(1, 16)  OutScaling=2^-10  DoSatur=off
  Discrete Derivative1 : simulink/Discrete/Discrete Derivative  gainval=1.0  ICPrevScaledInput=0.0  OutMin=[]  OutMax=[]  OutDataType=fixdt(1, 16)  OutScaling=2^-10  DoSatur=off
  Discrete Derivative2 : simulink/Discrete/Discrete Derivative  gainval=1.0  ICPrevScaledInput=0.0  OutMin=[]  OutMax=[]  OutDataType=fixdt(1, 16)  OutScaling=2^-10  DoSatur=off
  Matrix Multiply : Product  Multiplication=Matrix(*)
  Mux1 : Mux  Inputs=3
  Mux2 : Mux  Inputs=2
  Mux3 : Mux  Inputs=3
  Reshape1 : Reshape  OutputDimensionality=Column vector (2-D)
  Reshape3 : Reshape  OutputDimensionality=Column vector (2-D)
  Reshape4 : Reshape  OutputDimensionality=Column vector (2-D)
  Subtract{4..8} (5 alike) : Sum  Inputs=-+
  Terminator : Terminator
  u : Outport
  wires:
  Mux2/1 -> Matrix Multiply/2
  Reshape1/1 -> Mux2/1
  Mux1/1 -> Reshape1/1
  Reshape3/1 -> Mux2/2
  Reshape4/1 -> u/1
  Matrix Multiply/1 -> Reshape4/1
  Constant2/1 -> Matrix Multiply/1
  Mux3/1 -> Reshape3/1
  Demux1/2 -> Discrete Derivative1/1, Subtract4/1
  Demux/2 -> Subtract4/2
  Demux1/3 -> Discrete Derivative2/1, Calculate Error/1(Unwrapped Angle)
  Discrete Derivative1/1 -> Subtract6/1
  Demux/4 -> Subtract7/2
  Data Store Read13/1 -> Demux/1
  Demux/1 -> Subtract5/2
  Discrete Derivative/1 -> Subtract7/1
  Data Store Read1/1 -> Demux1/1
  Demux/5 -> Subtract6/2
  Demux/3 -> Calculate Error/2(Unwrapped Angle1)
  Demux/7 -> Terminator/1
  Discrete Derivative2/1 -> Subtract8/1
  Demux1/1 -> Discrete Derivative/1, Subtract5/1
  Demux/6 -> Subtract8/2
  Subtract5/1 -> Mux1/1
  Subtract4/1 -> Mux1/2
  Calculate Error/1(Attitude Error) -> Mux1/3
  Subtract7/1 -> Mux3/1
  Subtract6/1 -> Mux3/2
  Subtract8/1 -> Mux3/3

== system Template_v4_1_0_2024b_Jetson/3 - Control/Default LQR Control (BLUE) ==
  Action Port : ActionPort  ActionPortLabel=elseif(u1 == 2)
  Calculate Error : Subsystem
  Constant2 : Constant  Value=-K_BLUE
  Data Store Read1 : DataStoreRead  DataStoreName=BLUE_Path  IndexOptions=Index vector (dialog)  Indices=1  OutputSizes=1
  Data Store Read2 : DataStoreRead  DataStoreName=BLUE_Measured_States  IndexOptions=Index vector (dialog)  Indices=1  OutputSizes=1
  Demux : Demux  Outputs=[1,1,1,1,1,1,3]
  Demux1 : Demux  Outputs=3
  Discrete Derivative : simulink/Discrete/Discrete Derivative  gainval=1.0  ICPrevScaledInput=0.0  OutMin=[]  OutMax=[]  OutDataType=fixdt(1, 16)  OutScaling=2^-10  DoSatur=off
  Discrete Derivative1 : simulink/Discrete/Discrete Derivative  gainval=1.0  ICPrevScaledInput=0.0  OutMin=[]  OutMax=[]  OutDataType=fixdt(1, 16)  OutScaling=2^-10  DoSatur=off
  Discrete Derivative2 : simulink/Discrete/Discrete Derivative  gainval=1.0  ICPrevScaledInput=0.0  OutMin=[]  OutMax=[]  OutDataType=fixdt(1, 16)  OutScaling=2^-10  DoSatur=off
  Matrix Multiply : Product  Multiplication=Matrix(*)
  Mux : Mux  Inputs=3
  Mux1 : Mux  Inputs=2
  Mux2 : Mux  Inputs=3
  Reshape1 : Reshape  OutputDimensionality=Column vector (2-D)
  Reshape2 : Reshape  OutputDimensionality=Column vector (2-D)
  Reshape4 : Reshape  OutputDimensionality=Column vector (2-D)
  Subtract{4..8} (5 alike) : Sum  Inputs=-+
  Terminator : Terminator
  u : Outport
  wires:
  Calculate Error/1(Attitude Error) -> Mux/3
  Subtract6/1 -> Mux2/2
  Matrix Multiply/1 -> Reshape4/1
  Mux2/1 -> Reshape2/1
  Reshape4/1 -> u/1
  Mux/1 -> Reshape1/1
  Subtract5/1 -> Mux/1
  Reshape2/1 -> Mux1/2
  Mux1/1 -> Matrix Multiply/2
  Subtract7/1 -> Mux2/1
  Constant2/1 -> Matrix Multiply/1
  Subtract4/1 -> Mux/2
  Subtract8/1 -> Mux2/3
  Reshape1/1 -> Mux1/1
  Demux/2 -> Subtract4/2
  Demux/4 -> Subtract7/2
  Demux/7 -> Terminator/1
  Demux/1 -> Subtract5/2
  Data Store Read1/1 -> Demux1/1
  Discrete Derivative2/1 -> Subtract8/1
  Demux1/3 -> Discrete Derivative2/1, Calculate Error/1(Unwrapped Angle)
  Discrete Derivative/1 -> Subtract7/1
  Demux/3 -> Calculate Error/2(Unwrapped Angle1)
  Demux1/2 -> Discrete Derivative1/1, Subtract4/1
  Demux/6 -> Subtract8/2
  Demux/5 -> Subtract6/2
  Data Store Read2/1 -> Demux/1
  Demux1/1 -> Discrete Derivative/1, Subtract5/1
  Discrete Derivative1/1 -> Subtract6/1

== system Template_v4_1_0_2024b_Jetson/3 - Control/Default LQR Control (RED) ==
  Action Port : ActionPort  ActionPortLabel=elseif(u1 == 2)
  Calculate Error : Subsystem
  Constant2 : Constant  Value=-K_RED
  Data Store Read1 : DataStoreRead  DataStoreName=RED_Path  IndexOptions=Index vector (dialog)  Indices=1  OutputSizes=1
  Data Store Read13 : DataStoreRead  DataStoreName=RED_Measured_States  IndexOptions=Index vector (dialog)  Indices=1  OutputSizes=1
  Demux : Demux  Outputs=[1,1,1,1,1,1,3]
  Demux1 : Demux  Outputs=3
  Discrete Derivative : simulink/Discrete/Discrete Derivative  gainval=1.0  ICPrevScaledInput=0.0  OutMin=[]  OutMax=[]  OutDataType=fixdt(1, 16)  OutScaling=2^-10  DoSatur=off
  Discrete Derivative1 : simulink/Discrete/Discrete Derivative  gainval=1.0  ICPrevScaledInput=0.0  OutMin=[]  OutMax=[]  OutDataType=fixdt(1, 16)  OutScaling=2^-10  DoSatur=off
  Discrete Derivative2 : simulink/Discrete/Discrete Derivative  gainval=1.0  ICPrevScaledInput=0.0  OutMin=[]  OutMax=[]  OutDataType=fixdt(1, 16)  OutScaling=2^-10  DoSatur=off
  Display : Display
  Matrix Multiply : Product  Multiplication=Matrix(*)
  Mux1 : Mux  Inputs=3
  Mux2 : Mux  Inputs=2
  Mux3 : Mux  Inputs=3
  Reshape2 : Reshape  OutputDimensionality=Column vector (2-D)
  Reshape3 : Reshape  OutputDimensionality=Column vector (2-D)
  Reshape4 : Reshape  OutputDimensionality=Column vector (2-D)
  Subtract{4..8} (5 alike) : Sum  Inputs=-+
  Terminator : Terminator
  u : Outport
  wires:
  Subtract5/1 -> Mux1/1
  Mux2/1 -> Matrix Multiply/2
  Reshape3/1 -> Mux2/2
  Mux1/1 -> Reshape2/1
  Matrix Multiply/1 -> Reshape4/1
  Reshape4/1 -> u/1
  Subtract7/1 -> Mux3/1
  Reshape2/1 -> Mux2/1
  Mux3/1 -> Reshape3/1
  Constant2/1 -> Matrix Multiply/1
  Subtract4/1 -> Mux1/2
  Subtract8/1 -> Mux3/3
  Calculate Error/1(Attitude Error) -> Mux1/3
  Subtract6/1 -> Mux3/2
  Demux1/1 -> Discrete Derivative/1, Subtract5/1
  Discrete Derivative/1 -> Subtract7/1
  Demux1/3 -> Discrete Derivative2/1, Calculate Error/1(Unwrapped Angle)
  Discrete Derivative1/1 -> Subtract6/1
  Demux/5 -> Subtract6/2
  Demux/3 -> Calculate Error/2(Unwrapped Angle1)
  Demux/7 -> Terminator/1
  Data Store Read1/1 -> Demux1/1
  Demux/2 -> Subtract4/2
  Demux/1 -> Subtract5/2
  Demux/4 -> Subtract7/2
  Demux1/2 -> Discrete Derivative1/1, Subtract4/1
  Discrete Derivative2/1 -> Subtract8/1
  Data Store Read13/1 -> Display/1, Demux/1
  Demux/6 -> Subtract8/2

== system Template_v4_1_0_2024b_Jetson/3 - Control/Default PD (ARM) ==
  Action Port : ActionPort  ActionPortLabel=if(u1 == 1 )
  Constant7 : Constant
  Data Store Read2 : DataStoreRead  DataStoreName=ARM_Path  IndexOptions=Index vector (dialog)  Indices=1  OutputSizes=1
  Data Store Read4 : DataStoreRead  DataStoreName=isSim  IndexOptions=Index vector (dialog)  Indices=1  OutputSizes=1
  Data Store Write12 : DataStoreWrite  DataStoreName=ARM_Control_Mode  IndexOptions=Index vector (dialog)  Indices=1  OutputSizes=1
  Demux : Demux  Outputs=3
  "If 'simMode' set to '1', then this is a simulation and the dynamics will be simulated. Otherwise, this is an experiment, and the simulation will not be run." : If  IfExpression=u1 == 1
  Merge3 : Merge
  Merge4 : Merge
  Merge5 : Merge
  Mux : Mux  Inputs=3
  Passthrough for Experiment : Subsystem  TreatAsAtomicUnit=on
  Scope : Scope
  Simulated Position Controller : Subsystem  TreatAsAtomicUnit=on
  u : Outport
  wires:
  Passthrough for Experiment/3(q3_command) -> Merge5/2
  Data Store Read4/1 -> "If 'simMode' set to '1', then this is a simulation and the dynamics will be simulated. Otherwise, this is an experiment, and the simulation will not be run."/1
  Demux/3 -> Passthrough for Experiment/3(q3_desired), Simulated Position Controller/3(q3_desired)
  Simulated Position Controller/1(q1_command) -> Merge3/1
  Simulated Position Controller/3(q3_command) -> Merge5/1
  "If 'simMode' set to '1', then this is a simulation and the dynamics will be simulated. Otherwise, this is an experiment, and the simulation will not be run."/1 -> Simulated Position Controller/Action
  Demux/2 -> Passthrough for Experiment/2(q2_desired), Simulated Position Controller/2(q2_desired)
  Passthrough for Experiment/2(q2_command) -> Merge4/2
  Simulated Position Controller/2(q2_command) -> Merge4/1
  Constant7/1 -> Data Store Write12/1
  Passthrough for Experiment/1(q1_command) -> Merge3/2
  Demux/1 -> Passthrough for Experiment/1(q1_desired), Simulated Position Controller/1(q1_desired)
  "If 'simMode' set to '1', then this is a simulation and the dynamics will be simulated. Otherwise, this is an experiment, and the simulation will not be run."/2 -> Passthrough for Experiment/Action
  Merge3/1 -> Mux/1
  Merge4/1 -> Mux/2
  Merge5/1 -> Mux/3
  Mux/1 -> Scope/1, u/1
  Data Store Read2/1 -> Demux/1

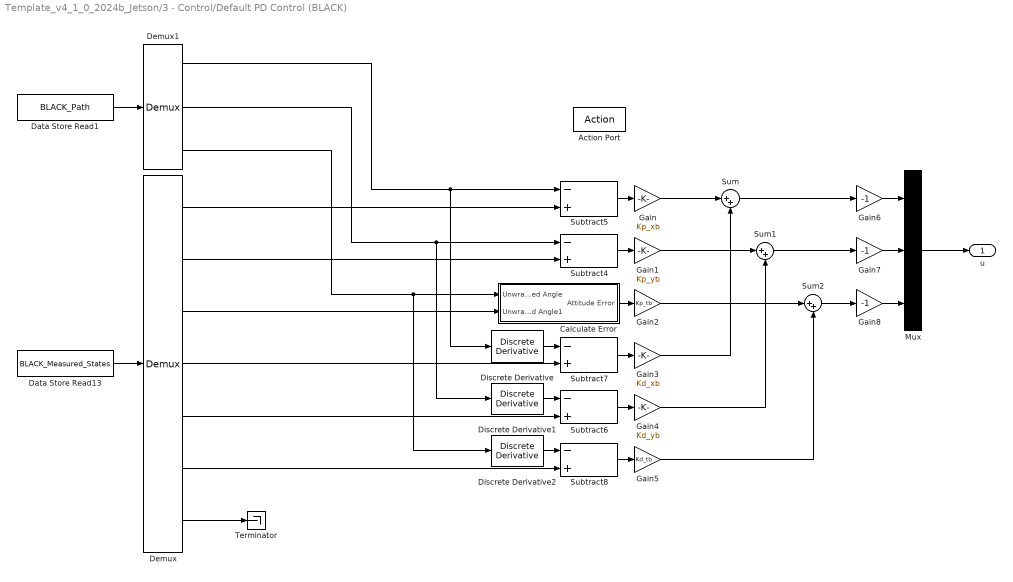
== system Template_v4_1_0_2024b_Jetson/3 - Control/Default PD Control (BLACK) ==
  Action Port : ActionPort  ActionPortLabel=if(u1 == 1 )
  Calculate Error : Subsystem
  Data Store Read1 : DataStoreRead  DataStoreName=BLACK_Path  IndexOptions=Index vector (dialog)  Indices=1  OutputSizes=1
  Data Store Read13 : DataStoreRead  DataStoreName=BLACK_Measured_States  IndexOptions=Index vector (dialog)  Indices=1  OutputSizes=1
  Demux : Demux  Outputs=[1,1,1,1,1,1,3]
  Demux1 : Demux  Outputs=3
  Discrete Derivative : simulink/Discrete/Discrete Derivative  gainval=1.0  ICPrevScaledInput=0.0  OutMin=[]  OutMax=[]  OutDataType=fixdt(1, 16)  OutScaling=2^-10  DoSatur=off
  Discrete Derivative1 : simulink/Discrete/Discrete Derivative  gainval=1.0  ICPrevScaledInput=0.0  OutMin=[]  OutMax=[]  OutDataType=fixdt(1, 16)  OutScaling=2^-10  DoSatur=off
  Discrete Derivative2 : simulink/Discrete/Discrete Derivative  gainval=1.0  ICPrevScaledInput=0.0  OutMin=[]  OutMax=[]  OutDataType=fixdt(1, 16)  OutScaling=2^-10  DoSatur=off
  Gain : Gain  Gain=Kp_xb
  Gain1 : Gain  Gain=Kp_yb
  Gain2 : Gain  Gain=Kp_tb
  Gain3 : Gain  Gain=Kd_xb
  Gain4 : Gain  Gain=Kd_yb
  Gain5 : Gain  Gain=Kd_tb
  Gain6 : Gain  Gain=-1
  Gain7 : Gain  Gain=-1
  Gain8 : Gain  Gain=-1
  Mux : Mux  Inputs=3
  Subtract{4..8} (5 alike) : Sum  Inputs=-+
  Sum : Sum  Inputs=|++
  Sum1 : Sum  Inputs=|++
  Sum2 : Sum  Inputs=|++
  Terminator : Terminator
  u : Outport
  wires:
  Demux/6 -> Subtract8/2
  Subtract8/1 -> Gain5/1
  Gain8/1 -> Mux/3
  Discrete Derivative2/1 -> Subtract8/1
  Gain1/1 -> Sum1/1
  Subtract5/1 -> Gain/1
  Discrete Derivative1/1 -> Subtract6/1
  Subtract6/1 -> Gain4/1
  Demux/2 -> Subtract4/2
  Demux/1 -> Subtract5/2
  Sum1/1 -> Gain7/1
  Demux/4 -> Subtract7/2
  Demux1/3 -> Discrete Derivative2/1, Calculate Error/1(Unwrapped Angle)
  Sum/1 -> Gain6/1
  Subtract4/1 -> Gain1/1
  Demux/3 -> Calculate Error/2(Unwrapped Angle1)
  Subtract7/1 -> Gain3/1
  Gain3/1 -> Sum/2
  Mux/1 -> u/1
  Gain4/1 -> Sum1/2
  Demux1/2 -> Discrete Derivative1/1, Subtract4/1
  Gain/1 -> Sum/1
  Demux/5 -> Subtract6/2
  Gain5/1 -> Sum2/2
  Discrete Derivative/1 -> Subtract7/1
  Demux1/1 -> Discrete Derivative/1, Subtract5/1
  Sum2/1 -> Gain8/1
  Calculate Error/1(Attitude Error) -> Gain2/1
  Gain7/1 -> Mux/2
  Gain6/1 -> Mux/1
  Gain2/1 -> Sum2/1
  Data Store Read13/1 -> Demux/1
  Demux/7 -> Terminator/1
  Data Store Read1/1 -> Demux1/1

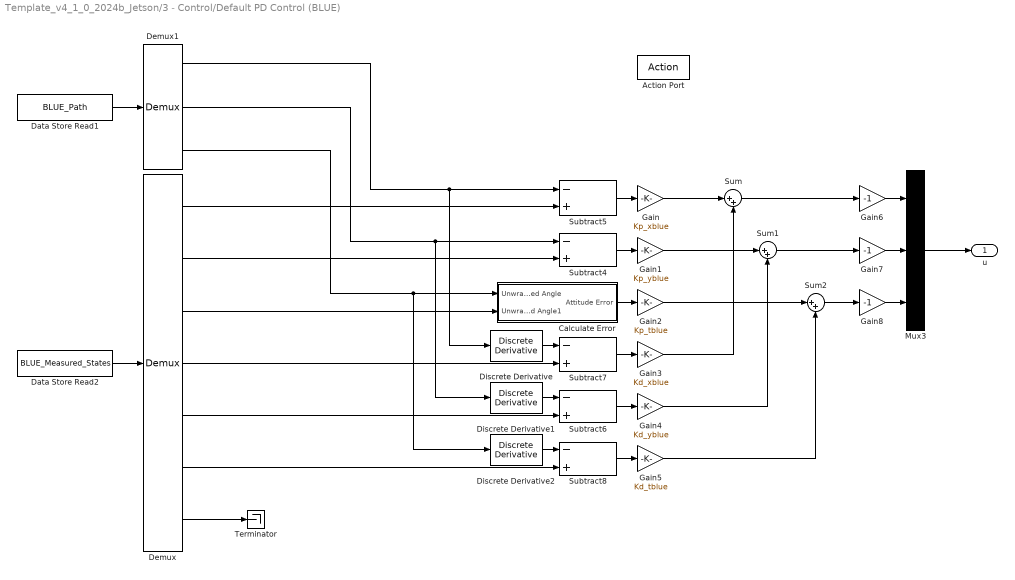
== system Template_v4_1_0_2024b_Jetson/3 - Control/Default PD Control (BLUE) ==
  Action Port : ActionPort  ActionPortLabel=if(u1 == 1 )
  Calculate Error : Subsystem
  Data Store Read1 : DataStoreRead  DataStoreName=BLUE_Path  IndexOptions=Index vector (dialog)  Indices=1  OutputSizes=1
  Data Store Read2 : DataStoreRead  DataStoreName=BLUE_Measured_States  IndexOptions=Index vector (dialog)  Indices=1  OutputSizes=1
  Demux : Demux  Outputs=[1,1,1,1,1,1,3]
  Demux1 : Demux  Outputs=3
  Discrete Derivative : simulink/Discrete/Discrete Derivative  gainval=1.0  ICPrevScaledInput=0.0  OutMin=[]  OutMax=[]  OutDataType=fixdt(1, 16)  OutScaling=2^-10  DoSatur=off
  Discrete Derivative1 : simulink/Discrete/Discrete Derivative  gainval=1.0  ICPrevScaledInput=0.0  OutMin=[]  OutMax=[]  OutDataType=fixdt(1, 16)  OutScaling=2^-10  DoSatur=off
  Discrete Derivative2 : simulink/Discrete/Discrete Derivative  gainval=1.0  ICPrevScaledInput=0.0  OutMin=[]  OutMax=[]  OutDataType=fixdt(1, 16)  OutScaling=2^-10  DoSatur=off
  Gain : Gain  Gain=Kp_xblue
  Gain1 : Gain  Gain=Kp_yblue
  Gain2 : Gain  Gain=Kp_tblue
  Gain3 : Gain  Gain=Kd_xblue
  Gain4 : Gain  Gain=Kd_yblue
  Gain5 : Gain  Gain=Kd_tblue
  Gain6 : Gain  Gain=-1
  Gain7 : Gain  Gain=-1
  Gain8 : Gain  Gain=-1
  Mux3 : Mux  Inputs=3
  Subtract{4..8} (5 alike) : Sum  Inputs=-+
  Sum : Sum  Inputs=|++
  Sum1 : Sum  Inputs=|++
  Sum2 : Sum  Inputs=|++
  Terminator : Terminator
  u : Outport
  wires:
  Sum/1 -> Gain6/1
  Mux3/1 -> u/1
  Gain3/1 -> Sum/2
  Sum2/1 -> Gain8/1
  Gain5/1 -> Sum2/2
  Sum1/1 -> Gain7/1
  Gain6/1 -> Mux3/1
  Gain4/1 -> Sum1/2
  Gain1/1 -> Sum1/1
  Gain2/1 -> Sum2/1
  Gain8/1 -> Mux3/3
  Gain7/1 -> Mux3/2
  Gain/1 -> Sum/1
  Demux1/1 -> Discrete Derivative/1, Subtract5/1
  Discrete Derivative/1 -> Subtract7/1
  Demux1/3 -> Discrete Derivative2/1, Calculate Error/1(Unwrapped Angle)
  Discrete Derivative1/1 -> Subtract6/1
  Demux/5 -> Subtract6/2
  Demux/3 -> Calculate Error/2(Unwrapped Angle1)
  Demux/7 -> Terminator/1
  Data Store Read1/1 -> Demux1/1
  Demux/2 -> Subtract4/2
  Demux/1 -> Subtract5/2
  Demux/4 -> Subtract7/2
  Demux1/2 -> Discrete Derivative1/1, Subtract4/1
  Discrete Derivative2/1 -> Subtract8/1
  Data Store Read2/1 -> Demux/1
  Demux/6 -> Subtract8/2
  Subtract5/1 -> Gain/1
  Subtract4/1 -> Gain1/1
  Calculate Error/1(Attitude Error) -> Gain2/1
  Subtract7/1 -> Gain3/1
  Subtract6/1 -> Gain4/1
  Subtract8/1 -> Gain5/1

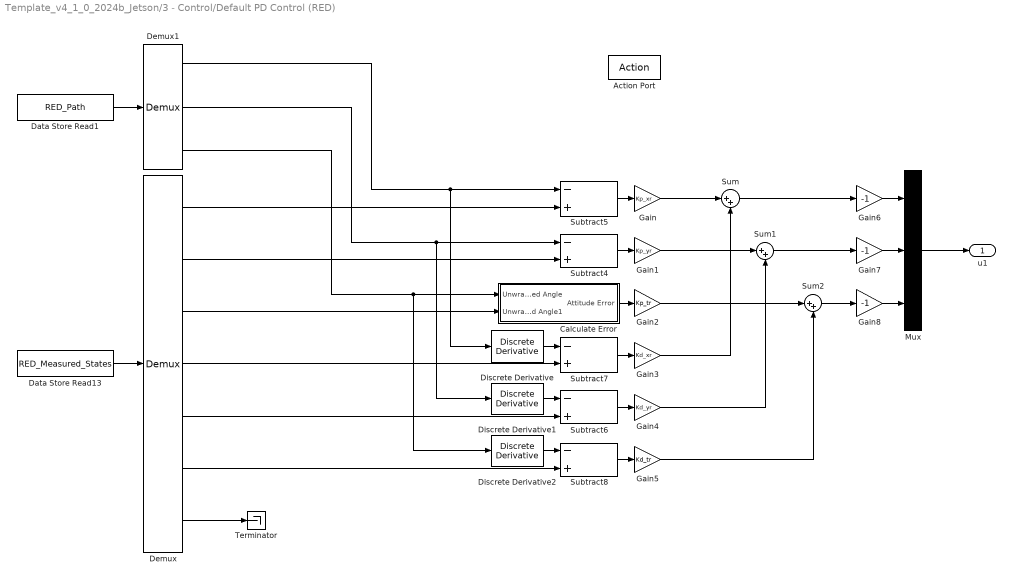
== system Template_v4_1_0_2024b_Jetson/3 - Control/Default PD Control (RED) ==
  Action Port : ActionPort  ActionPortLabel=if(u1 == 1 )
  Calculate Error : Subsystem
  Data Store Read1 : DataStoreRead  DataStoreName=RED_Path  IndexOptions=Index vector (dialog)  Indices=1  OutputSizes=1
  Data Store Read13 : DataStoreRead  DataStoreName=RED_Measured_States  IndexOptions=Index vector (dialog)  Indices=1  OutputSizes=1
  Demux : Demux  Outputs=[1,1,1,1,1,1,3]
  Demux1 : Demux  Outputs=3
  Discrete Derivative : simulink/Discrete/Discrete Derivative  gainval=1.0  ICPrevScaledInput=0.0  OutMin=[]  OutMax=[]  OutDataType=fixdt(1, 16)  OutScaling=2^-10  DoSatur=off
  Discrete Derivative1 : simulink/Discrete/Discrete Derivative  gainval=1.0  ICPrevScaledInput=0.0  OutMin=[]  OutMax=[]  OutDataType=fixdt(1, 16)  OutScaling=2^-10  DoSatur=off
  Discrete Derivative2 : simulink/Discrete/Discrete Derivative  gainval=1.0  ICPrevScaledInput=0.0  OutMin=[]  OutMax=[]  OutDataType=fixdt(1, 16)  OutScaling=2^-10  DoSatur=off
  Gain : Gain  Gain=Kp_xr
  Gain1 : Gain  Gain=Kp_yr
  Gain2 : Gain  Gain=Kp_tr
  Gain3 : Gain  Gain=Kd_xr
  Gain4 : Gain  Gain=Kd_yr
  Gain5 : Gain  Gain=Kd_tr
  Gain6 : Gain  Gain=-1
  Gain7 : Gain  Gain=-1
  Gain8 : Gain  Gain=-1
  Mux : Mux  Inputs=3
  Subtract{4..8} (5 alike) : Sum  Inputs=-+
  Sum : Sum  Inputs=|++
  Sum1 : Sum  Inputs=|++
  Sum2 : Sum  Inputs=|++
  Terminator : Terminator
  u1 : Outport
  wires:
  Gain6/1 -> Mux/1
  Gain8/1 -> Mux/3
  Gain1/1 -> Sum1/1
  Sum/1 -> Gain6/1
  Gain5/1 -> Sum2/2
  Gain3/1 -> Sum/2
  Sum1/1 -> Gain7/1
  Mux/1 -> u1/1
  Gain4/1 -> Sum1/2
  Sum2/1 -> Gain8/1
  Gain/1 -> Sum/1
  Gain7/1 -> Mux/2
  Gain2/1 -> Sum2/1
  Demux1/2 -> Discrete Derivative1/1, Subtract4/1
  Demux/2 -> Subtract4/2
  Demux1/3 -> Discrete Derivative2/1, Calculate Error/1(Unwrapped Angle)
  Discrete Derivative1/1 -> Subtract6/1
  Demux/4 -> Subtract7/2
  Data Store Read13/1 -> Demux/1
  Demux/1 -> Subtract5/2
  Discrete Derivative/1 -> Subtract7/1
  Data Store Read1/1 -> Demux1/1
  Demux/5 -> Subtract6/2
  Demux/3 -> Calculate Error/2(Unwrapped Angle1)
  Demux/7 -> Terminator/1
  Discrete Derivative2/1 -> Subtract8/1
  Demux1/1 -> Discrete Derivative/1, Subtract5/1
  Demux/6 -> Subtract8/2
  Subtract5/1 -> Gain/1
  Subtract4/1 -> Gain1/1
  Calculate Error/1(Attitude Error) -> Gain2/1
  Subtract7/1 -> Gain3/1
  Subtract6/1 -> Gain4/1
  Subtract8/1 -> Gain5/1

== system Template_v4_1_0_2024b_Jetson/3 - Control/Disable Control (ARM) ==
  Action Port : ActionPort  ActionPortLabel=else
  Constant7 : Constant  Value=0
  Data Store Write12 : DataStoreWrite  DataStoreName=ARM_Control_Mode  IndexOptions=Index vector (dialog)  Indices=1  OutputSizes=1
  Mux : Mux  Inputs=3
  Zero : Constant  Value=0  OutDataTypeStr=Inherit: Inherit via back propagation
  Out1 : Outport
  wires:
  Mux/1 -> Out1/1
  Zero/1 -> Mux/3, Mux/1, Mux/2
  Constant7/1 -> Data Store Write12/1

== system Template_v4_1_0_2024b_Jetson/3 - Control/Disable Thrusters (BLACK) ==
  Action Port : ActionPort  ActionPortLabel=else
  Mux : Mux  Inputs=3
  Zero : Constant  Value=0  OutDataTypeStr=Inherit: Inherit via back propagation
  Out1 : Outport
  wires:
  Zero/1 -> Mux/3, Mux/1, Mux/2
  Mux/1 -> Out1/1

== system Template_v4_1_0_2024b_Jetson/3 - Control/Disable Thrusters (BLUE) ==
  Action Port : ActionPort  ActionPortLabel=else
  Mux : Mux  Inputs=3
  Zero : Constant  Value=0  OutDataTypeStr=Inherit: Inherit via back propagation
  Out1 : Outport
  wires:
  Zero/1 -> Mux/3, Mux/1, Mux/2
  Mux/1 -> Out1/1

== system Template_v4_1_0_2024b_Jetson/3 - Control/Disable Thrusters (RED) ==
  Action Port : ActionPort  ActionPortLabel=else
  Mux : Mux  Inputs=3
  Zero : Constant  Value=0  OutDataTypeStr=Inherit: Inherit via back propagation
  u : Outport
  wires:
  Zero/1 -> Mux/3, Mux/1, Mux/2
  Mux/1 -> u/1

== system Template_v4_1_0_2024b_Jetson/Check Connection/Change BLACK Behavior ==
  Action Port : ActionPort  ActionPortLabel=if(u1 == 2 & u2 == 0)
  Constant1 : Constant  OutDataTypeStr=int32
  UDP Send : nvidiaSharedBlocks/UDP Send  remoteURL='255.255.255.255'  remotePort=33002  localURL='0.0.0.0'  localPortSource=Automatically determine  localPort=-1  sampletime=-1  blockPlatform=NVIDIA  separateLengthPort=0
      settings: LibrarySourceBlock=nvidiaNetworklib/UDP Send
  wires:
  Constant1/1 -> UDP Send/1

== system Template_v4_1_0_2024b_Jetson/Check Connection/Change BLUE Behavior ==
  Action Port : ActionPort  ActionPortLabel=if(u1 == 3 & u2 == 0)
  Constant1 : Constant  OutDataTypeStr=int32
  UDP Send : nvidiaSharedBlocks/UDP Send  remoteURL='255.255.255.255'  remotePort=33003  localURL='0.0.0.0'  localPortSource=Automatically determine  localPort=-1  sampletime=-1  blockPlatform=NVIDIA  separateLengthPort=0
      settings: LibrarySourceBlock=nvidiaNetworklib/UDP Send
  wires:
  Constant1/1 -> UDP Send/1

== system Template_v4_1_0_2024b_Jetson/Check Connection/Change RED Behavior ==
  Action Port : ActionPort  ActionPortLabel=if(u1 == 1 & u2 == 0)
  Constant1 : Constant  OutDataTypeStr=int32
  UDP Send : nvidiaSharedBlocks/UDP Send  remoteURL='255.255.255.255'  remotePort=33001  localURL='0.0.0.0'  localPortSource=Automatically determine  localPort=-1  sampletime=-1  blockPlatform=NVIDIA  separateLengthPort=0
      settings: LibrarySourceBlock=nvidiaNetworklib/UDP Send
  wires:
  Constant1/1 -> UDP Send/1

== system Template_v4_1_0_2024b_Jetson/Debugger/Change BLACK Behavior ==
  Action Port : ActionPort  ActionPortLabel=if(u1 == 2 & u2 == 0)
  Data Type Conversion1 : DataTypeConversion  OutDataTypeStr=uint8  SaturateOnIntegerOverflow=off  RndMeth=Floor
  String Constant1 : StringConstant  String="\"Target: Hello\""
  String to ASCII1 : StringToASCII
  UDP Send1 : nvidiaSharedBlocks/UDP Send  remoteURL='255.255.255.255'  remotePort=55000  localURL='0.0.0.0'  localPortSource=Automatically determine  localPort=-1  sampletime=-1  blockPlatform=NVIDIA  separateLengthPort=0
      settings: LibrarySourceBlock=nvidiaNetworklib/UDP Send
  wires:
  Data Type Conversion1/1 -> UDP Send1/1
  String Constant1/1 -> String to ASCII1/1
  String to ASCII1/1 -> Data Type Conversion1/1

== system Template_v4_1_0_2024b_Jetson/Debugger/Change BLUE Behavior ==
  Action Port : ActionPort  ActionPortLabel=if(u1 == 3 & u2 == 0)
  Data Type Conversion2 : DataTypeConversion  OutDataTypeStr=uint8  SaturateOnIntegerOverflow=off  RndMeth=Floor
  String Constant2 : StringConstant  String="\"Obstacle: Hello\""
  String to ASCII2 : StringToASCII
  UDP Send2 : nvidiaSharedBlocks/UDP Send  remoteURL='255.255.255.255'  remotePort=55000  localURL='0.0.0.0'  localPortSource=Automatically determine  localPort=-1  sampletime=-1  blockPlatform=NVIDIA  separateLengthPort=0
      settings: LibrarySourceBlock=nvidiaNetworklib/UDP Send
  wires:
  Data Type Conversion2/1 -> UDP Send2/1
  String to ASCII2/1 -> Data Type Conversion2/1
  String Constant2/1 -> String to ASCII2/1

== system Template_v4_1_0_2024b_Jetson/Debugger/Change RED Behavior ==
  Action Port : ActionPort  ActionPortLabel=if(u1 == 1 & u2 == 0)
  Data Store Read : DataStoreRead  DataStoreName=RED_Logger  IndexOptions=Index vector (dialog)  Indices=1  OutputSizes=1
  Data Type Conversion : DataTypeConversion  OutDataTypeStr=uint8  SaturateOnIntegerOverflow=off  RndMeth=Floor
  String to ASCII : StringToASCII
  UDP Send3 : nvidiaSharedBlocks/UDP Send  remoteURL='255.255.255.255'  remotePort=55000  localURL='0.0.0.0'  localPortSource=Automatically determine  localPort=-1  sampletime=-1  blockPlatform=NVIDIA  separateLengthPort=0
      settings: LibrarySourceBlock=nvidiaNetworklib/UDP Send
  wires:
  Data Store Read/1 -> String to ASCII/1
  Data Type Conversion/1 -> UDP Send3/1
  String to ASCII/1 -> Data Type Conversion/1

== system Template_v4_1_0_2024b_Jetson/Float Code/Enable Pucks ==
  Action Port : ActionPort  ActionPortLabel=if(u1 == 0)
  Data Store Read1 : DataStoreRead  DataStoreName=Float_State  IndexOptions=Index vector (dialog)  Indices=1  OutputSizes=1
  GPIO Write1 : MainLibrary/Jetson Functions/GPIO Write  gpioPin=428  pinDirection=1
      settings: SourceProductName=SPOT Custom Library
  wires:
  Data Store Read1/1 -> GPIO Write1/1
